simulink model "cordic_cells"  (Simulink 6.6)
settings: Solver=VariableStepDiscrete  StartTime=0.0  StopTime=1  RelTol=1e-3
StopFcn:
  | figure(1)
  | hold off
  | plot([0 1], [0 0],'k:');
  | hold on
  | plot([0 0], [-0.5 0.5],'k-');
  | plot([0 x_in_rot(1)], [0 0], 'r-','LineWidth',2);
  | plot([0 x_out_rot(1)], [0 y_out_rot(1)],'b-','LineWidth',2);
  | legend('X axis', 'Y axis', 'Input Vector','Output Vector',4);
  | xlabel('X');
  | ylabel('Y');
  | title('Rotation Cell');
  | axis([0 1 -0.5 0.5]);
  | axis equal
  | 
  | figure(2)
  | hold off
  | plot([0 1], [0 0],'k:');
  | hold on
  | plot([0 0], [-0.5 0.5],'k-');
  | plot([0 x_in_vec(1)], [0 y_in_vec(1)], 'r-','LineWidth',2);
  | plot([0 x_out_vec(1)], [0 y_out_vec(1)],'b-','LineWidth',2);
  | legend('X axis', 'Y axis', 'Input Vector','Output Vector',4);
  | xlabel('X');
  | ylabel('Y');
  | title('Vectoring Cell');
  | axis([0 1 -0.5 0.5]);
  | axis equal
libraries: xbsIndex_r4 x31
settings Model: Creator=lcrockett  LastModifiedBy=lcrockett
settings OptimizationCC: InlineParams=on

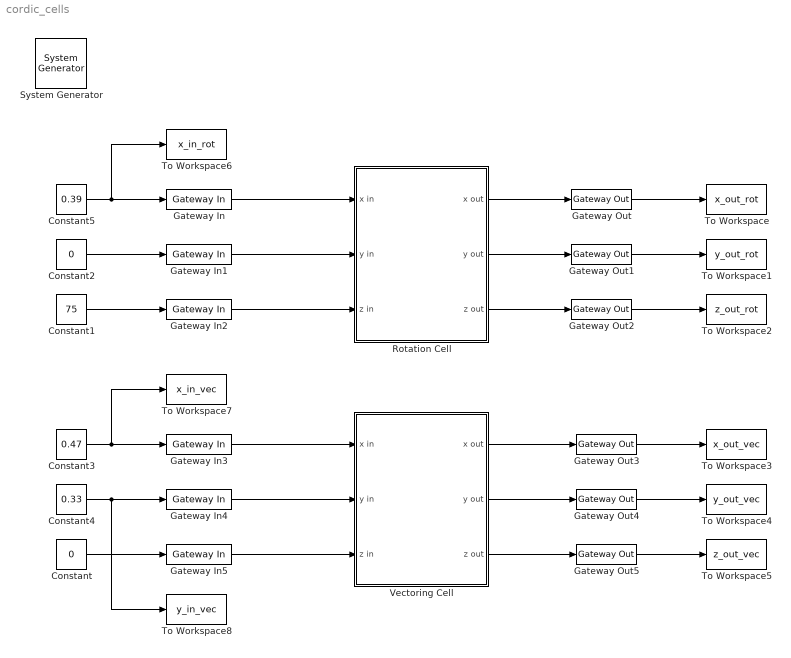
== system cordic_cells ==
  " System Generator" : xbsIndex_r4/ System Generator  Tag=genX  SystemSampleTime=-1  xilinxfamily=virtex2p  part=xc2vp30  speed=-7  package=ff896  synthesis_tool=XST  clock_wrapper=Clock Enables  directory=./netlist  testbench=off  simulink_period=1  sysclk_period=100  dcm_input_clock_period=100  incr_netlist=off  trim_vbits=Everywhere in SubSystem  dbl_ovrd=According to Block Masks  core_generation=According to Block Masks  run_coregen=off  deprecated_control=off  eval_field=0  block_type=sysgen
      settings: block_version=10.1.2
  Constant : Constant  Value=0  SampleTime=1
  Constant1 : Constant  Value=75  SampleTime=1
  Constant2 : Constant  Value=0  SampleTime=1
  Constant3 : Constant  Value=0.47  SampleTime=1
  Constant4 : Constant  Value=0.33  SampleTime=1
  Constant5 : Constant  Value=0.39  SampleTime=1
  Gateway In{,1..5} (6 alike) : xbsIndex_r4/Gateway In  arith_type="Signed  (2's comp)"  n_bits=15  bin_pt=12  quantization="Round  (unbiased: +/- Inf)"  overflow=Saturate  period=1  dbl_ovrd=off  timing_constraint=None  locs_specified=off  LOCs={}  block_type=gatewayin
      settings: infoedit="Gateway in block.  Converts inputs of type Simulink integer, double and fixed point to  Xilinx fixed point type.<P><P>Hardware notes:  In hardware these blocks become top level input ports."  block_version=10.1.2
  Gateway Out{,1..5} (6 alike) : xbsIndex_r4/Gateway Out  hdl_port=on  timing_constraint=None  locs_specified=off  LOCs={}  block_type=gatewayout
      settings: infoedit="Gateway out block.  Converts Xilinx fixed point inputs into ouputs of type Simulink integer, double, or fixed point.<P><P>Hardware notes:  In hardware these blocks become top level output ports or are discarded, depending on how they are configured."  block_version=10.1.2
  Rotation Cell : Subsystem
  To Workspace : ToWorkspace  VariableName=x_out_rot  SampleTime=-1  SaveFormat=Array
  To Workspace1 : ToWorkspace  VariableName=y_out_rot  SampleTime=-1  SaveFormat=Array
  To Workspace2 : ToWorkspace  VariableName=z_out_rot  SampleTime=-1  SaveFormat=Array
  To Workspace3 : ToWorkspace  VariableName=x_out_vec  SampleTime=-1  SaveFormat=Array
  To Workspace4 : ToWorkspace  VariableName=y_out_vec  SampleTime=-1  SaveFormat=Array
  To Workspace5 : ToWorkspace  VariableName=z_out_vec  SampleTime=-1  SaveFormat=Array
  To Workspace6 : ToWorkspace  VariableName=x_in_rot  SampleTime=-1  SaveFormat=Array
  To Workspace7 : ToWorkspace  VariableName=x_in_vec  SampleTime=-1  SaveFormat=Array
  To Workspace8 : ToWorkspace  VariableName=y_in_vec  SampleTime=-1  SaveFormat=Array
  Vectoring Cell : Subsystem
  wires:
  Gateway In/1 -> Rotation Cell/1(x in)
  Gateway In1/1 -> Rotation Cell/2(y in)
  Gateway In2/1 -> Rotation Cell/3(z in)
  Gateway In3/1 -> Vectoring Cell/1(x in)
  Gateway In4/1 -> Vectoring Cell/2(y in)
  Gateway In5/1 -> Vectoring Cell/3(z in)
  Constant/1 -> Gateway In5/1
  Constant1/1 -> Gateway In2/1
  Constant2/1 -> Gateway In1/1
  Constant3/1 -> Gateway In3/1, To Workspace7/1
  Constant4/1 -> Gateway In4/1, To Workspace8/1
  Constant5/1 -> Gateway In/1, To Workspace6/1
  Rotation Cell/1(x out) -> Gateway Out/1
  Rotation Cell/3(z out) -> Gateway Out2/1
  Rotation Cell/2(y out) -> Gateway Out1/1
  Vectoring Cell/1(x out) -> Gateway Out3/1
  Vectoring Cell/2(y out) -> Gateway Out4/1
  Vectoring Cell/3(z out) -> Gateway Out5/1
  Gateway Out/1 -> To Workspace/1
  Gateway Out1/1 -> To Workspace1/1
  Gateway Out2/1 -> To Workspace2/1
  Gateway Out3/1 -> To Workspace3/1
  Gateway Out4/1 -> To Workspace4/1
  Gateway Out5/1 -> To Workspace5/1

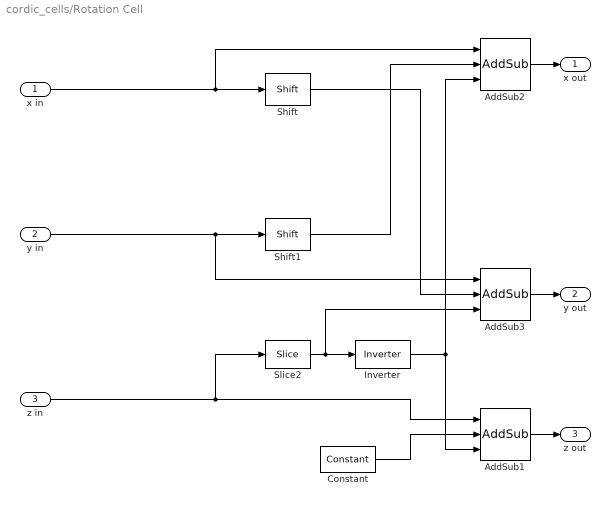
== system cordic_cells/Rotation Cell ==
  x in : Inport
  y in : Inport  Port=2
  z in : Inport  Port=3
  AddSub1 : xbsIndex_r4/AddSub  mode=Addition or Subtraction  use_carryin=off  use_carryout=off  en=off  latency=0  precision=User Defined  arith_type="Signed  (2's comp)"  n_bits=20  bin_pt=12  quantization=Truncate  overflow=Wrap  dbl_ovrd=off  use_behavioral_HDL=on  pipelined=off  use_rpm=on  block_type=addsub
      settings: xl_area=[0, 0, 0, 0, 0, 0, 0]  block_version=VER_STRING_GOES_HERE
  AddSub2 : xbsIndex_r4/AddSub  mode=Addition or Subtraction  use_carryin=off  use_carryout=off  en=off  latency=0  precision=User Defined  arith_type="Signed  (2's comp)"  n_bits=15  bin_pt=12  quantization=Truncate  overflow=Wrap  dbl_ovrd=off  use_behavioral_HDL=on  pipelined=off  use_rpm=on  block_type=addsub
      settings: xl_area=[0, 0, 0, 0, 0, 0, 0]  block_version=VER_STRING_GOES_HERE
  AddSub3 : xbsIndex_r4/AddSub  mode=Addition or Subtraction  use_carryin=off  use_carryout=off  en=off  latency=0  precision=User Defined  arith_type="Signed  (2's comp)"  n_bits=15  bin_pt=12  quantization=Truncate  overflow=Wrap  dbl_ovrd=off  use_behavioral_HDL=on  pipelined=off  use_rpm=on  block_type=addsub
      settings: xl_area=[0, 0, 0, 0, 0, 0, 0]  block_version=VER_STRING_GOES_HERE
  Constant : xbsIndex_r4/Constant  arith_type=Signed (2's comp)  const=atand(2^-0)  n_bits=20  bin_pt=12  explicit_period=off  period=1  equ=P=C  opselect=C  inp2=PCIN>>17  opr=+  inp1=P  carry=CIN  dbl_ovrd=off  block_type=constant
      settings: block_version=10.1.2
  Inverter : xbsIndex_r4/Inverter  en=off  latency=0  dbl_ovrd=off  block_type=inv
      settings: block_version=10.1.2
  Shift : xbsIndex_r4/Shift  shift_dir=Right  shift_bits=0  en=off  latency=0  precision=User Defined  arith_type="Signed  (2's comp)"  n_bits=15  bin_pt=12  quantization=Truncate  overflow=Wrap  dbl_ovrd=off  block_type=shift
      settings: xl_area=[0, 0, 0, 0, 0, 0, 0]  block_version=VER_STRING_GOES_HERE
  Shift1 : xbsIndex_r4/Shift  shift_dir=Right  shift_bits=0  en=off  latency=0  precision=User Defined  arith_type="Signed  (2's comp)"  n_bits=15  bin_pt=12  quantization=Truncate  overflow=Wrap  dbl_ovrd=off  block_type=shift
      settings: xl_area=[0, 0, 0, 0, 0, 0, 0]  block_version=VER_STRING_GOES_HERE
  Slice2 : xbsIndex_r4/Slice  nbits=1  boolean_output=on  mode=Upper Bit Location + Width  bit1=0  base1=MSB of Input  bit0=0  base0=LSB of Input  dbl_ovrd=off  block_type=slice
      settings: infoedit="Extracts a given range of bits from each input sample and presents it at the output.  The output type is ordinarily unsigned with binary point at zero, but can be Boolean when the slice is one bit wide.<P><P>Hardware notes: In hardware this block costs nothing."  block_version=VER_STRING_GOES_HERE
  x out : Outport
  y out : Outport  Port=2
  z out : Outport  Port=3
  wires:
  x in/1 -> AddSub2/1, Shift/1
  y in/1 -> AddSub3/1, Shift1/1
  Shift1/1 -> AddSub2/2
  Shift/1 -> AddSub3/2
  AddSub2/1 -> x out/1
  AddSub3/1 -> y out/1
  z in/1 -> AddSub1/1, Slice2/1
  Constant/1 -> AddSub1/2
  Slice2/1 -> Inverter/1, AddSub3/3
  AddSub1/1 -> z out/1
  Inverter/1 -> AddSub1/3, AddSub2/3

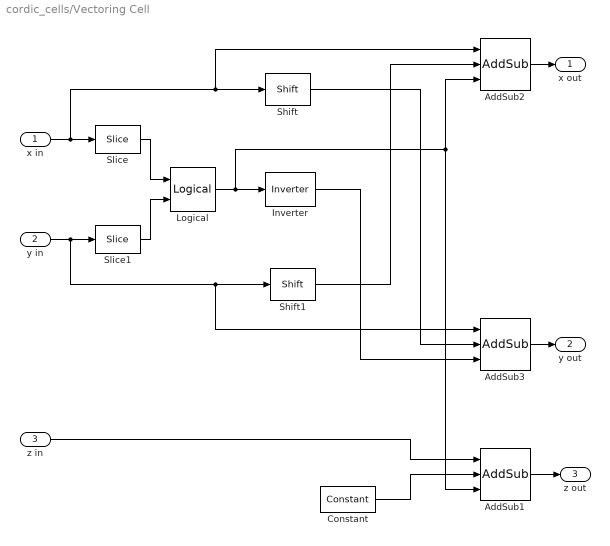
== system cordic_cells/Vectoring Cell ==
  x in : Inport
  y in : Inport  Port=2
  z in : Inport  Port=3
  AddSub1 : xbsIndex_r4/AddSub  mode=Addition or Subtraction  use_carryin=off  use_carryout=off  en=off  latency=0  precision=User Defined  arith_type="Signed  (2's comp)"  n_bits=20  bin_pt=12  quantization=Truncate  overflow=Wrap  dbl_ovrd=off  use_behavioral_HDL=on  pipelined=off  use_rpm=on  block_type=addsub
      settings: xl_area=[0, 0, 0, 0, 0, 0, 0]  block_version=VER_STRING_GOES_HERE
  AddSub2 : xbsIndex_r4/AddSub  mode=Addition or Subtraction  use_carryin=off  use_carryout=off  en=off  latency=0  precision=User Defined  arith_type="Signed  (2's comp)"  n_bits=15  bin_pt=12  quantization=Truncate  overflow=Wrap  dbl_ovrd=off  use_behavioral_HDL=on  pipelined=off  use_rpm=on  block_type=addsub
      settings: xl_area=[0, 0, 0, 0, 0, 0, 0]  block_version=VER_STRING_GOES_HERE
  AddSub3 : xbsIndex_r4/AddSub  mode=Addition or Subtraction  use_carryin=off  use_carryout=off  en=off  latency=0  precision=User Defined  arith_type="Signed  (2's comp)"  n_bits=15  bin_pt=12  quantization=Truncate  overflow=Wrap  dbl_ovrd=off  use_behavioral_HDL=on  pipelined=off  use_rpm=on  block_type=addsub
      settings: xl_area=[0, 0, 0, 0, 0, 0, 0]  block_version=VER_STRING_GOES_HERE
  Constant : xbsIndex_r4/Constant  arith_type=Signed (2's comp)  const=atand(2^-0)  n_bits=20  bin_pt=12  explicit_period=off  period=1  equ=P=C  opselect=C  inp2=PCIN>>17  opr=+  inp1=P  carry=CIN  dbl_ovrd=off  block_type=constant
      settings: block_version=10.1.2
  Inverter : xbsIndex_r4/Inverter  en=off  latency=0  dbl_ovrd=off  block_type=inv
      settings: xl_area=[0, 0, 0, 0, 0, 0, 0]  block_version=VER_STRING_GOES_HERE
  Logical : xbsIndex_r4/Logical  logical_function=XOR  inputs=2  en=off  latency=0  precision=Full  arith_type=Unsigned  n_bits=1  bin_pt=0  align_bp=on  dbl_ovrd=off  block_type=logical
      settings: xl_area=[0, 0, 0, 0, 0, 0, 0]  block_version=VER_STRING_GOES_HERE
  Shift : xbsIndex_r4/Shift  shift_dir=Right  shift_bits=0  en=off  latency=0  precision=User Defined  arith_type="Signed  (2's comp)"  n_bits=15  bin_pt=12  quantization=Truncate  overflow=Wrap  dbl_ovrd=off  block_type=shift
      settings: xl_area=[0, 0, 0, 0, 0, 0, 0]  block_version=VER_STRING_GOES_HERE
  Shift1 : xbsIndex_r4/Shift  shift_dir=Right  shift_bits=0  en=off  latency=0  precision=User Defined  arith_type="Signed  (2's comp)"  n_bits=15  bin_pt=12  quantization=Truncate  overflow=Wrap  dbl_ovrd=off  block_type=shift
      settings: xl_area=[0, 0, 0, 0, 0, 0, 0]  block_version=VER_STRING_GOES_HERE
  Slice : xbsIndex_r4/Slice  nbits=1  boolean_output=on  mode=Upper Bit Location + Width  bit1=0  base1=MSB of Input  bit0=0  base0=LSB of Input  dbl_ovrd=off  block_type=slice
      settings: infoedit="Extracts a given range of bits from each input sample and presents it at the output.  The output type is ordinarily unsigned with binary point at zero, but can be Boolean when the slice is one bit wide.<P><P>Hardware notes: In hardware this block costs nothing."  block_version=VER_STRING_GOES_HERE
  Slice1 : xbsIndex_r4/Slice  nbits=1  boolean_output=on  mode=Upper Bit Location + Width  bit1=0  base1=MSB of Input  bit0=0  base0=LSB of Input  dbl_ovrd=off  block_type=slice
      settings: infoedit="Extracts a given range of bits from each input sample and presents it at the output.  The output type is ordinarily unsigned with binary point at zero, but can be Boolean when the slice is one bit wide.<P><P>Hardware notes: In hardware this block costs nothing."  block_version=VER_STRING_GOES_HERE
  x out : Outport
  y out : Outport  Port=2
  z out : Outport  Port=3
  wires:
  x in/1 -> AddSub2/1, Shift/1, Slice/1
  y in/1 -> AddSub3/1, Shift1/1, Slice1/1
  Slice/1 -> Logical/1
  Slice1/1 -> Logical/2
  Logical/1 -> Inverter/1, AddSub2/3, AddSub1/3
  Shift1/1 -> AddSub2/2
  Shift/1 -> AddSub3/2
  Inverter/1 -> AddSub3/3
  AddSub2/1 -> x out/1
  AddSub3/1 -> y out/1
  z in/1 -> AddSub1/1
  Constant/1 -> AddSub1/2
  AddSub1/1 -> z out/1
